simulink model "APP"  (R2020b)
settings: configuration reference "cs_ert" (kept outside this file)
settings Model: DataDictionary=APP.sldd  EnableAccessToBaseWorkspace=off  Creator=zhoutinglin  LastModifiedBy=zhoutinglin
settings ConfigSetRef: SourceName=cs_ert

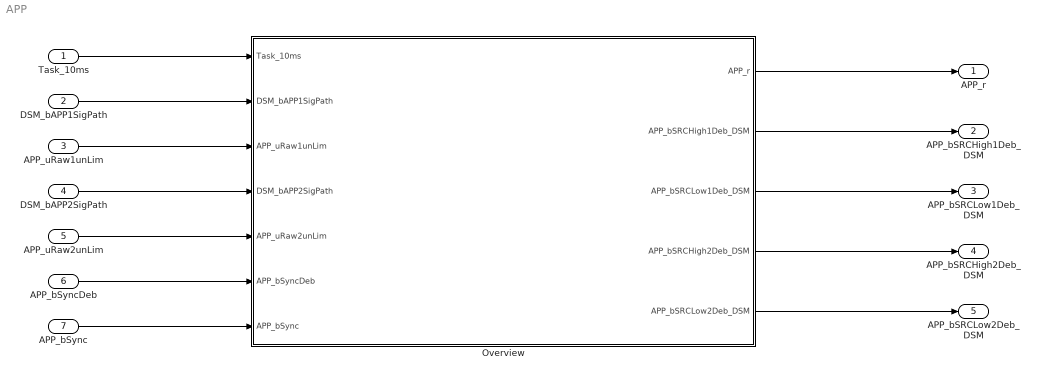
== system APP ==
  Task_10ms : Inport  OutputFunctionCall=on
  DSM_bAPP1SigPath : Inport  Port=2
  APP_uRaw1unLim : Inport  Port=3
  DSM_bAPP2SigPath : Inport  Port=4
  APP_uRaw2unLim : Inport  Port=5
  APP_bSyncDeb : Inport  Port=6
  APP_bSync : Inport  Port=7
  Overview : Subsystem
  APP_r : Outport
  APP_bSRCHigh1Deb_DSM : Outport  Port=2
  APP_bSRCLow1Deb_DSM : Outport  Port=3
  APP_bSRCHigh2Deb_DSM : Outport  Port=4
  APP_bSRCLow2Deb_DSM : Outport  Port=5
  wires:
  Task_10ms/1 -> Overview/1(Task_10ms)
  DSM_bAPP1SigPath/1 -> Overview/2(DSM_bAPP1SigPath)
  APP_uRaw1unLim/1 -> Overview/3(APP_uRaw1unLim)
  DSM_bAPP2SigPath/1 -> Overview/4(DSM_bAPP2SigPath)
  APP_uRaw2unLim/1 -> Overview/5(APP_uRaw2unLim)
  APP_bSyncDeb/1 -> Overview/6(APP_bSyncDeb)
  APP_bSync/1 -> Overview/7(APP_bSync)
  Overview/1(APP_r) -> APP_r/1
  Overview/2(APP_bSRCHigh1Deb_DSM) -> APP_bSRCHigh1Deb_DSM/1
  Overview/3(APP_bSRCLow1Deb_DSM) -> APP_bSRCLow1Deb_DSM/1
  Overview/4(APP_bSRCHigh2Deb_DSM) -> APP_bSRCHigh2Deb_DSM/1
  Overview/5(APP_bSRCLow2Deb_DSM) -> APP_bSRCLow2Deb_DSM/1

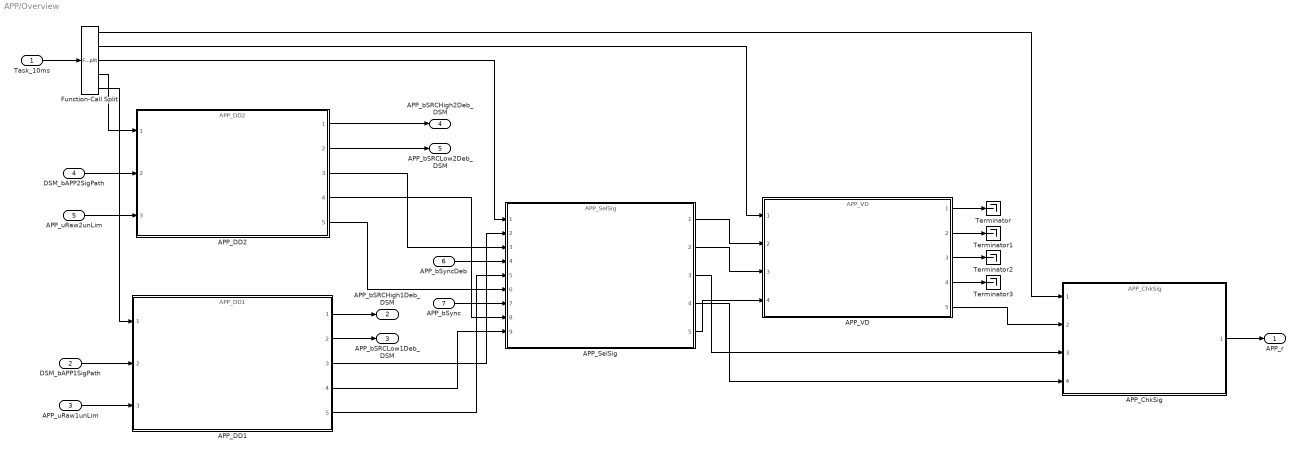
== system APP/Overview ==
  Task_10ms : Inport
  DSM_bAPP1SigPath : Inport  Port=2
  APP_uRaw1unLim : Inport  Port=3
  DSM_bAPP2SigPath : Inport  Port=4
  APP_uRaw2unLim : Inport  Port=5
  APP_bSyncDeb : Inport  Port=6
  APP_bSync : Inport  Port=7
  APP_ChkSig : ModelReference  ModelNameDialog=APP_ChkSig  SimulationMode=Normal  ScheduleRates=on  ModelReferenceVersion=1.53
  APP_DD1 : ModelReference  ModelNameDialog=APP_DD1  SimulationMode=Normal  ScheduleRates=on  ModelReferenceVersion=1.60
  APP_DD2 : ModelReference  ModelNameDialog=APP_DD2  SimulationMode=Normal  ScheduleRates=on  ModelReferenceVersion=1.53
  APP_SelSig : ModelReference  ModelNameDialog=APP_SelSig  SimulationMode=Normal  ScheduleRates=on  ModelReferenceVersion=1.53
  APP_VD : ModelReference  ModelNameDialog=APP_VD  SimulationMode=Normal  ScheduleRates=on  ModelReferenceVersion=1.55
  Function-Call Split : FunctionCallSplit  IconShape=distinctive  NumOutputPorts=5  OutputPortLayout=default
  Terminator{,1..3} (4 alike) : Terminator
  APP_r : Outport  VectorParamsAs1DForOutWhenUnconnected=off
  APP_bSRCHigh1Deb_DSM : Outport  Port=2  VectorParamsAs1DForOutWhenUnconnected=off
  APP_bSRCLow1Deb_DSM : Outport  Port=3  VectorParamsAs1DForOutWhenUnconnected=off
  APP_bSRCHigh2Deb_DSM : Outport  Port=4  VectorParamsAs1DForOutWhenUnconnected=off
  APP_bSRCLow2Deb_DSM : Outport  Port=5  VectorParamsAs1DForOutWhenUnconnected=off
  wires:
  APP_ChkSig/1 -> APP_r/1
  APP_DD1/1 -> APP_bSRCHigh1Deb_DSM/1
  APP_DD1/2 -> APP_bSRCLow1Deb_DSM/1
  APP_DD2/1 -> APP_bSRCHigh2Deb_DSM/1
  APP_DD2/2 -> APP_bSRCLow2Deb_DSM/1
  APP_VD/1 -> Terminator/1
  APP_VD/2 -> Terminator1/1
  APP_VD/3 -> Terminator2/1
  APP_VD/4 -> Terminator3/1
  DSM_bAPP1SigPath/1 -> APP_DD1/2
  APP_uRaw1unLim/1 -> APP_DD1/3
  DSM_bAPP2SigPath/1 -> APP_DD2/2
  APP_uRaw2unLim/1 -> APP_DD2/3
  APP_DD2/3 -> APP_SelSig/3
  APP_DD2/4 -> APP_SelSig/8
  APP_DD2/5 -> APP_SelSig/6
  APP_bSyncDeb/1 -> APP_SelSig/4
  APP_bSync/1 -> APP_SelSig/7
  APP_VD/5 -> APP_ChkSig/2
  APP_SelSig/4 -> APP_ChkSig/4
  APP_SelSig/1 -> APP_VD/2
  APP_SelSig/3 -> APP_ChkSig/3
  APP_SelSig/5 -> APP_VD/4
  APP_SelSig/2 -> APP_VD/3
  APP_DD1/3 -> APP_SelSig/2
  APP_DD1/4 -> APP_SelSig/9
  APP_DD1/5 -> APP_SelSig/5
  Task_10ms/1 -> Function-Call Split/1
  Function-Call Split/5 -> APP_DD1/1
  Function-Call Split/4 -> APP_DD2/1
  Function-Call Split/3 -> APP_SelSig/1
  Function-Call Split/2 -> APP_VD/1
  Function-Call Split/1 -> APP_ChkSig/1
